simulink model "chap9_1sim"  (R2015a)
settings: Solver=ode45  StartTime=0.0  StopTime=10.0  RelTol=1e-3
settings Model: Creator=zhr  LastModifiedBy=zhr

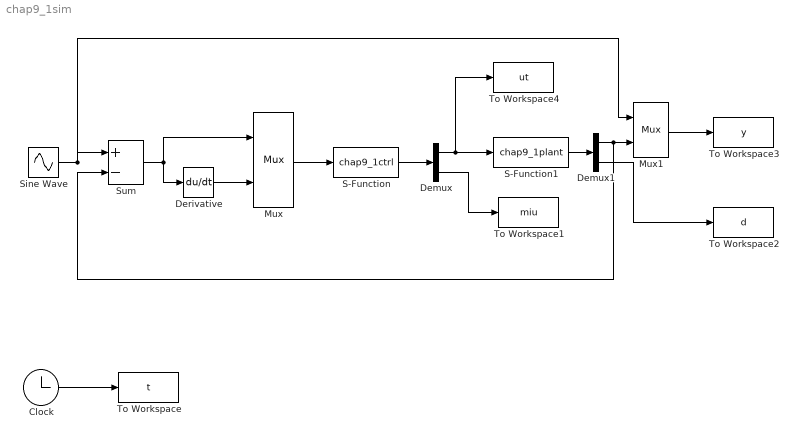
== system chap9_1sim ==
  Clock : Clock
  Demux : Demux  Outputs=2
  Demux1 : Demux  Outputs=2
  Derivative : Derivative
  Mux : Mux  Inputs=2
  Mux1 : Mux  Inputs=2
  S-Function : S-Function  FunctionName=chap9_1ctrl
  S-Function1 : S-Function  FunctionName=chap9_1plant
  Sine Wave : Sin  SampleTime=0
  Sum : Sum  Inputs=|+-
  To Workspace : ToWorkspace  VariableName=t  SampleTime=-1
  To Workspace1 : ToWorkspace  VariableName=miu  SampleTime=-1
  To Workspace2 : ToWorkspace  VariableName=d  SampleTime=-1
  To Workspace3 : ToWorkspace  VariableName=y  SampleTime=-1
  To Workspace4 : ToWorkspace  VariableName=ut  SampleTime=-1
  wires:
  Clock/1 -> To Workspace/1
  Sine Wave/1 -> Mux1/1, Sum/1
  Sum/1 -> Derivative/1, Mux/1
  Derivative/1 -> Mux/2
  Mux/1 -> S-Function/1
  S-Function/1 -> Demux/1
  Demux/1 -> To Workspace4/1, S-Function1/1
  Demux/2 -> To Workspace1/1
  S-Function1/1 -> Demux1/1
  Demux1/1 -> Sum/2, Mux1/2
  Demux1/2 -> To Workspace2/1
  Mux1/1 -> To Workspace3/1
